simulink subsystem "decoder_8b10b"  (R2022b)
settings: Solver=VariableStepAuto  StartTime=0.0  StopTime=10.0  RelTol=1e-3
settings Model: Creator=Ali-Laptop  LastModifiedBy=Ali-Laptop

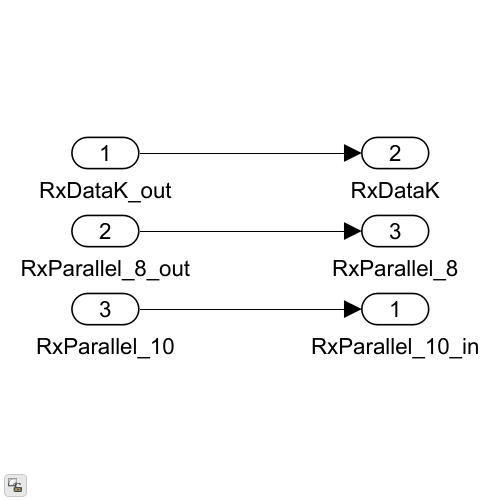
[thumbnail: Simulink's stored preview of the top-level diagram]
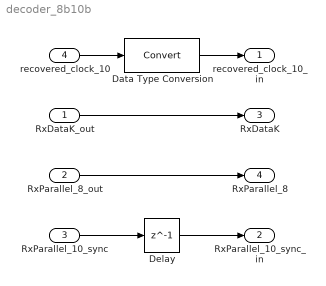
== system decoder_8b10b ==
  RxDataK_out : Inport
  RxParallel_8_out : Inport  Port=2
  RxParallel_10_sync : Inport  Port=3
  recovered_clock_10 : Inport  Port=4
  Data Type Conversion : DataTypeConversion  SaturateOnIntegerOverflow=off  RndMeth=Floor
  Delay : Delay  DelayLength=1
  recovered_clock_10_in : Outport
  RxParallel_10_sync_in : Outport  Port=2
  RxDataK : Outport  Port=3
  RxParallel_8 : Outport  Port=4
  wires:
  Data Type Conversion/1 -> recovered_clock_10_in/1
  recovered_clock_10/1 -> Data Type Conversion/1
  RxParallel_10_sync/1 -> Delay/1
  RxDataK_out/1 -> RxDataK/1
  RxParallel_8_out/1 -> RxParallel_8/1
  Delay/1 -> RxParallel_10_sync_in/1
